simulink model "model_autopilot_expanded"  (R2019a)
settings: Solver=VariableStepAuto  StartTime=0.0  StopTime=sim_time  RelTol=1e-3
values from neighbouring files (symbols this model uses):
  C = [0  0  1  0; 0  0  0  1]    [kalman_variables.mat]
undefined symbols (not defined in the file or in its folder): A, B, g, k_d_phi, k_i_chi, k_p_chi, k_p_phi, V_g
libraries: simulink_extras x3
settings Model: Creator=gustavoo  LastModifiedBy=gustavoo
settings DebuggingCC: ArithmeticOperatorsInVariantConditions=warning

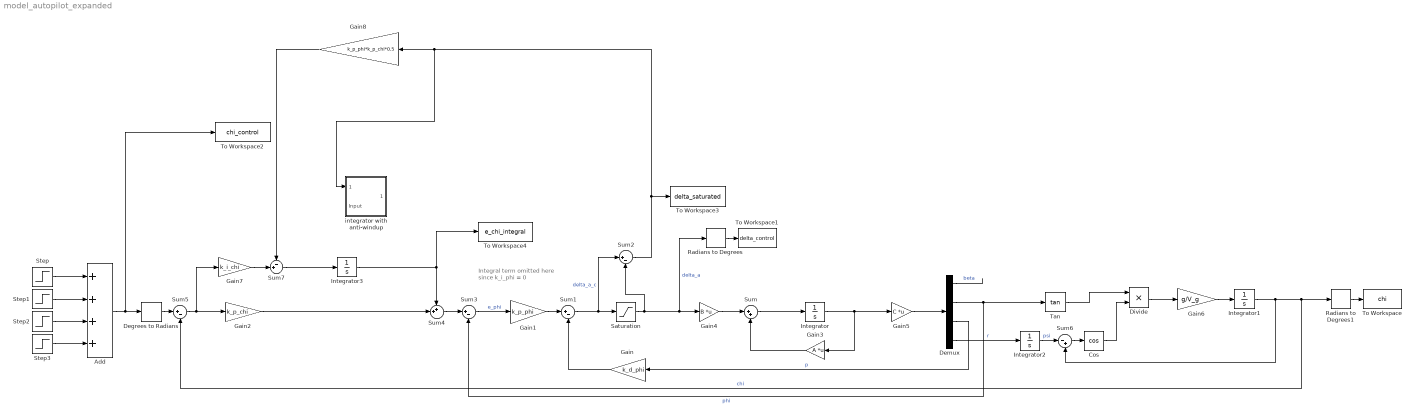
== system model_autopilot_expanded ==
  note: Integral term omitted here
      | since k_i_phi = 0
  Add : Sum  Inputs=++++
  Cos : Trigonometry  Operator=cos
  Degrees to Radians : simulink_extras/Transformations/Degrees to Radians
  Demux : Demux
  Divide : Product  Inputs=**
  Gain : Gain  Gain=k_d_phi
  Gain1 : Gain  Gain=k_p_phi
  Gain2 : Gain  Gain=k_p_chi
  Gain3 : Gain  Gain=A  Multiplication=Matrix(K*u)
  Gain4 : Gain  Gain=B  Multiplication=Matrix(K*u)
  Gain5 : Gain  Gain=C  Multiplication=Matrix(K*u)
  Gain6 : Gain  Gain=g/V_g
  Gain7 : Gain  Gain=k_i_chi
  Gain8 : Gain  Gain=k_p_phi*k_p_chi*0.5
  Integrator{,1..3} (4 alike) : Integrator
  Radians to Degrees : simulink_extras/Transformations/Radians to Degrees
  Radians to Degrees1 : simulink_extras/Transformations/Radians to Degrees
  Saturation : Saturate  UpperLimit=pi/6  LowerLimit=-pi/6
  Step : Step  Time=100  After=7.5  SampleTime=0
  Step1 : Step  Time=150  After=7.5  SampleTime=0
  Step2 : Step  Time=250  After=-15  SampleTime=0
  Step3 : Step  Time=300  After=0  SampleTime=0
  Sum : Sum  Inputs=|++
  Sum{1..3,5} (4 alike) : Sum  Inputs=|+-
  Sum4 : Sum  Inputs=++|
  Sum6 : Sum  Inputs=|-+
  Sum7 : Sum  Inputs=-+|
  Tan : Trigonometry  Operator=tan
  To Workspace : ToWorkspace  VariableName=chi  SaveFormat=Timeseries  SampleTime=-1
  To Workspace1 : ToWorkspace  VariableName=delta_control  SaveFormat=Timeseries  SampleTime=-1
  To Workspace2 : ToWorkspace  VariableName=chi_control  SaveFormat=Timeseries  SampleTime=-1
  To Workspace3 : ToWorkspace  VariableName=delta_saturated  SaveFormat=Timeseries  SampleTime=-1
  To Workspace4 : ToWorkspace  VariableName=e_chi_integral  SaveFormat=Timeseries  SampleTime=-1
  integrator with anti-windup : Subsystem
  wires:
  Sum1/1 -> Sum2/1, Saturation/1  "delta_a_c"
  Gain/1 -> Sum1/2
  Gain1/1 -> Sum1/1
  Sum3/1 -> Gain1/1  "e_phi"
  Sum4/1 -> Sum3/1
  Gain2/1 -> Sum4/2
  Sum5/1 -> Gain7/1, Gain2/1
  Integrator1/1 -> Sum6/2, Sum5/2, Radians to Degrees1/1  "chi"
  Saturation/1 -> Gain4/1, Radians to Degrees/1, Sum2/2  "delta_a"
  Degrees to Radians/1 -> Sum5/1
  Step1/1 -> Add/2
  Step/1 -> Add/1
  Step3/1 -> Add/4
  Step2/1 -> Add/3
  Add/1 -> To Workspace2/1, Degrees to Radians/1
  Radians to Degrees1/1 -> To Workspace/1
  Radians to Degrees/1 -> To Workspace1/1
  Sum2/1 -> integrator with anti-windup/1(delta_a), Gain8/1, To Workspace3/1
  Gain4/1 -> Sum/1
  Gain3/1 -> Sum/2
  Sum/1 -> Integrator/1
  Integrator/1 -> Gain3/1, Gain5/1
  Gain5/1 -> Demux/1
  Demux/1 -> ?  "beta"
  Demux/2 -> Tan/1, Sum3/2  "phi"
  Demux/3 -> Gain/1  "p"
  Demux/4 -> Integrator2/1  "r"
  Gain6/1 -> Integrator1/1
  Divide/1 -> Gain6/1
  Integrator2/1 -> Sum6/1  "psi"
  Tan/1 -> Divide/1
  Sum6/1 -> Cos/1
  Cos/1 -> Divide/2
  Gain7/1 -> Sum7/2
  Sum7/1 -> Integrator3/1
  Gain8/1 -> Sum7/1
  Integrator3/1 -> To Workspace4/1, Sum4/1

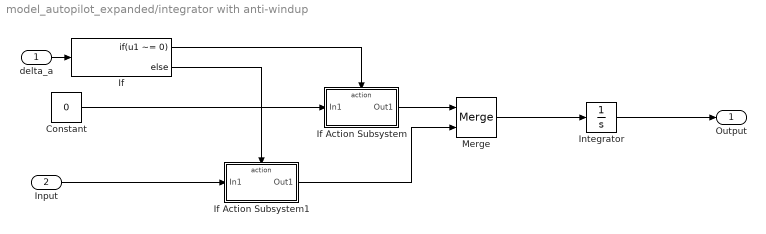
== system model_autopilot_expanded/integrator with anti-windup ==
  delta_a : Inport
  Input : Inport  Port=2
  Constant : Constant  Value=0
  If : If  IfExpression=u1 ~= 0
  If Action Subsystem : Subsystem  TreatAsAtomicUnit=on
  If Action Subsystem1 : Subsystem  TreatAsAtomicUnit=on
  Integrator : Integrator
  Merge : Merge
  Output : Outport
  wires:
  If/2 -> If Action Subsystem1/Action
  If/1 -> If Action Subsystem/Action
  If Action Subsystem1/1(Out1) -> Merge/2
  If Action Subsystem/1(Out1) -> Merge/1
  delta_a/1 -> If/1
  Constant/1 -> If Action Subsystem/1(In1)
  Input/1 -> If Action Subsystem1/1(In1)
  Merge/1 -> Integrator/1
  Integrator/1 -> Output/1

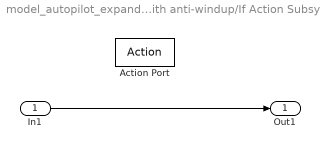
== system model_autopilot_expanded/integrator with anti-windup/If Action Subsystem ==
  In1 : Inport
  Action Port : ActionPort  ActionPortLabel=if(u1 ~= 0)
  Out1 : Outport
  wires:
  In1/1 -> Out1/1

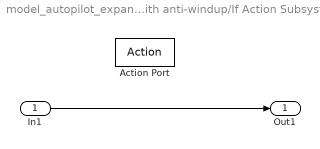
== system model_autopilot_expanded/integrator with anti-windup/If Action Subsystem1 ==
  In1 : Inport
  Action Port : ActionPort  ActionPortLabel=else
  Out1 : Outport
  wires:
  In1/1 -> Out1/1
